simulink library "desat_timer_logic_lib"  (R2018b)
settings: Solver=VariableStepAuto  StartTime=0.0  StopTime=10.0  RelTol=1e-3
undefined symbols (not defined in the file or in its folder): fswParams
settings Model: Creator=colem  LastModifiedBy=colem

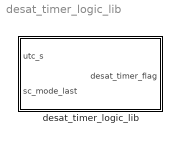
== system desat_timer_logic_lib ==
  desat_timer_logic_lib : Subsystem

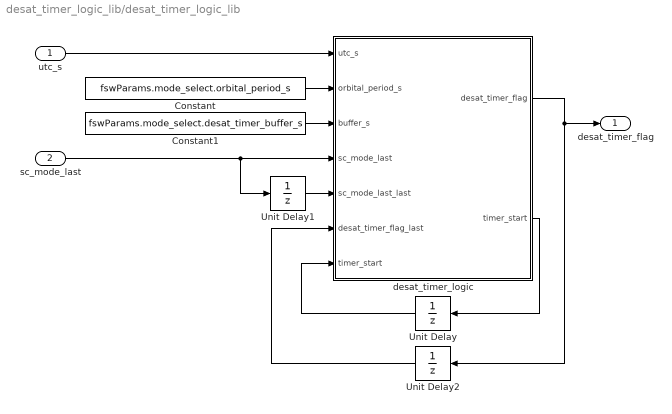
== system desat_timer_logic_lib/desat_timer_logic_lib ==
  utc_s : Inport
  sc_mode_last : Inport  Port=2
  Constant : Constant  Value=fswParams.mode_select.orbital_period_s  SampleTime=fswParams.sample_time_s
  Constant1 : Constant  Value=fswParams.mode_select.desat_timer_buffer_s  SampleTime=fswParams.sample_time_s
  Unit Delay : UnitDelay  SampleTime=fswParams.sample_time_s
  Unit Delay1 : UnitDelay  SampleTime=fswParams.sample_time_s
  Unit Delay2 : UnitDelay  SampleTime=fswParams.sample_time_s
  desat_timer_logic : MATLAB Function  TreatAsAtomicUnit=on
  desat_timer_flag : Outport
  wires:
  Unit Delay/1 -> desat_timer_logic/7("timer_start ")
  Constant1/1 -> desat_timer_logic/3(buffer_s)
  desat_timer_logic/2(timer_start) -> Unit Delay/1
  utc_s/1 -> desat_timer_logic/1(utc_s)
  desat_timer_logic/1(desat_timer_flag) -> Unit Delay2/1, desat_timer_flag/1
  Constant/1 -> desat_timer_logic/2(orbital_period_s)
  Unit Delay1/1 -> desat_timer_logic/5(sc_mode_last_last)
  sc_mode_last/1 -> Unit Delay1/1, desat_timer_logic/4(sc_mode_last)
  Unit Delay2/1 -> desat_timer_logic/6(desat_timer_flag_last)

== matlab function desat_timer_logic_lib/desat_timer_logic ==
  data: utc_s input; desat_timer_flag output; orbital_period_s input; buffer_s input; sc_mode_last input; sc_mode_last_last input; desat_timer_flag_last input; timer_start input; timer_start output
% Author: Cole Morgan

% This function ensures that desat mode / attitude stabilization mode last about an integer multiple
% of our orbital period. Once desat mode is tripped, the timer starts.
% This flag will go high until we are about one full orbital period from
% where we started. This way, since we are sun/nadir pointing, the pointing
% objective should be about the same as the beginning of desat mode, and
% the error to be corrected will be small. Ensures we sit in ASM mode once
% desat is done until about one orbit later.

function [desat_timer_flag, timer_start] = desat_timer(utc_s, orbital_period_s, buffer_s, sc_mode_last, sc_mode_last_last, ...
    desat_timer_flag_last, timer_start)

desat_timer_flag = desat_timer_flag_last;

if(sc_mode_last == 41.0)
    if(sc_mode_last_last ~= 41.0)
        % first iteration of desat mode
        timer_start = utc_s;
        
        desat_timer_flag = 1; % make sure to stay in ASM if not close to 
                          % the orbital period
    end
end
    
%     desat_timer_flag = 1; % make sure to stay in desat mode if not close to 
%                           % the orbital period 
  
if(desat_timer_flag == 1)
    delta_t_s = utc_s - timer_start; %seconds
    temp = mod(delta_t_s, orbital_period_s);
    if(temp < buffer_s  && delta_t_s > buffer_s)
        % check within buffer_s seconds of the orbital period.
        % also check that you are not just exiting instantly. NOTE: this
        % will guaruntee that a desat will not be shorter than buffer
        % seconds, but that is a very safe assumption anyway

        desat_timer_flag = 0; % allow to exit desat based on timer. wheel rpms
                              % checked elsewhere.
    end
end
end
